simulink model "Encode_To_DC"  (Simulink 8.6)
settings: Solver=VariableStepAuto  StartTime=0.0  StopTime=inf  RelTol=1e-3
libraries: hdlsllib x30, simulink x26, dspnetwork x2
settings Model: Creator=Oscar  LastModifiedBy=Oscar
settings DataIOCC: SaveFormat=Dataset  SignalLoggingSaveFormat=Dataset
settings OptimizationCC: ExpressionDepthLimit=128
settings DebuggingCC: UnderspecifiedInitializationDetection=Simplified  MergeDetectMultiDrivingBlocksExec=error  SolverPrmCheckMsg=none  FcnCallInpInsideContextMsg=EnableAllAsError  StateNameClashWarn=none
settings HardwareCC: ProdBitPerPointer=64  ProdLargestAtomicFloat=Float  ProdIntDivRoundTo=Zero  ProdEndianess=LittleEndian  ProdWordSize=64  ProdHWDeviceType=Intel->x86-64 (Windows64)
settings GRTTargetCC: GeneratePreprocessorConditionals=Use local settings  CombineOutputUpdateFcns=on  GRTInterface=off
settings ConfigComp: CovModelRefEnable=off

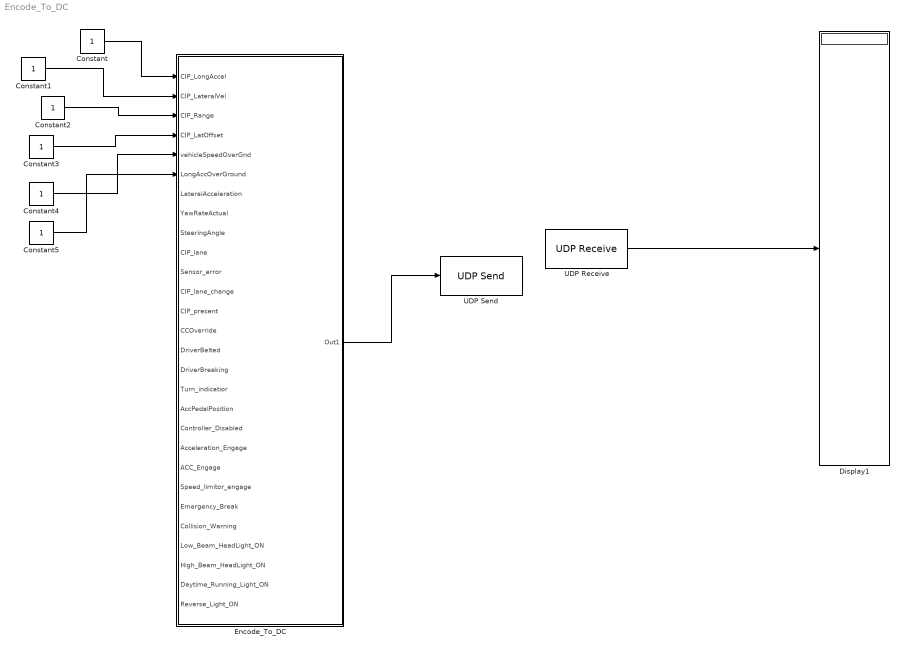
== system Encode_To_DC ==
  Constant{,1..5} (6 alike) : Constant
  Display1 : Display
      settings: Format=hex (Stored Integer)
  Encode_To_DC : Subsystem
  UDP Receive : dspnetwork/UDP Receive  localURL='0.0.0.0'  localPort=25000  remoteURL='localhost'  remotePort=-1  recvBufferSize=8192  dims=255  signalDatatype=uint16  isVarSize=on  showBlockingTime=off  blockingTime=0  sampletime=1
  UDP Send : dspnetwork/UDP Send  remoteURL='127.0.0.1'  remotePort=25000  localURL='0.0.0.0'  localPortSource=Automatically determine  localPort=-1  sampletime=-1  separateLengthPort=0
  wires:
  Encode_To_DC/1(Out1) -> UDP Send/1
  Constant/1 -> Encode_To_DC/1(CIP_LongAccel)
  UDP Receive/1 -> Display1/1
  Constant1/1 -> Encode_To_DC/2(CIP_LateralVel)
  Constant2/1 -> Encode_To_DC/3(CIP_Range)
  Constant3/1 -> Encode_To_DC/4(CIP_LatOffset)
  Constant4/1 -> Encode_To_DC/5(vehicleSpeedOverGnd)
  Constant5/1 -> Encode_To_DC/6(LongAccOverGround)

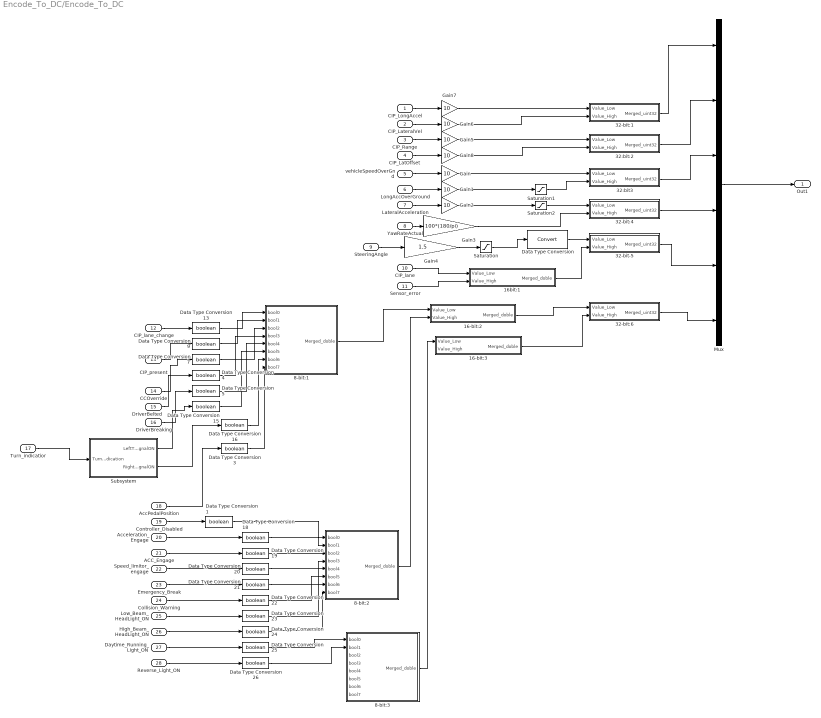
== system Encode_To_DC/Encode_To_DC ==
  CIP_LongAccel : Inport
  CIP_LateralVel : Inport  Port=2
  CIP_Range : Inport  Port=3
  CIP_LatOffset : Inport  Port=4
  vehicleSpeedOverGnd : Inport  Port=5
  LongAccOverGround : Inport  Port=6
  LateralAcceleration : Inport  Port=7
  YawRateActual : Inport  Port=8
  SteeringAngle : Inport  Port=9
  CIP_lane : Inport  Port=10
  Sensor_error : Inport  Port=11
  CIP_lane_change : Inport  Port=12
  CIP_present : Inport  Port=13
  CCOverride : Inport  Port=14
  DriverBelted : Inport  Port=15
  DriverBreaking : Inport  Port=16
  Turn_indicatior : Inport  Port=17
  AccPedalPosition : Inport  Port=18
  Controller_Disabled : Inport  Port=19
  Acceleration_Engage : Inport  Port=20
  ACC_Engage : Inport  Port=21
  Speed_limitor_engage : Inport  Port=22
  Emergency_Break : Inport  Port=23
  Collision_Warning : Inport  Port=24
  Low_Beam_HeadLight_ON : Inport  Port=25
  High_Beam_HeadLight_ON : Inport  Port=26
  Daytime_Running_Light_ON : Inport  Port=27
  Reverse_Light_ON : Inport  Port=28
  16-bit:2 : Subsystem
  16-bit:3 : Subsystem
  16bit:1 : Subsystem
  32-bit-5 : Subsystem
  32-bit:1 : Subsystem
  32-bit:4 : Subsystem
  32-bit:6 : Subsystem
  32:bit3 : Subsystem
  32:bit:2 : Subsystem
  8-bit:1 : Subsystem
  8-bit:2 : Subsystem
  8-bit:3 : Subsystem
  Data Type Conversion : DataTypeConversion
  Data Type Conversion{1,3..5,7,9,13,15..16,18..26} (18 alike) : DataTypeConversion  OutDataTypeStr=boolean  RndMeth=Nearest
  Gain{,1..2,5..8} (7 alike) : Gain  Gain=10
  Gain3 : Gain  Gain=100*(180/pi)
  Gain4 : Gain  Gain=1.5  OutMin=[-511]  OutMax=[512]  OutDataTypeStr=int16  SaturateOnIntegerOverflow=on
  Mux : Mux  Inputs=6
  Saturation : Saturate  UpperLimit=512  LowerLimit=-511
  Saturation1 : Saturate  UpperLimit=160  LowerLimit=-160
  Saturation2 : Saturate  UpperLimit=160  LowerLimit=-160
  Subsystem : Subsystem
  Out1 : Outport
  wires:
  LongAccOverGround/1 -> Gain1/1
  CIP_LateralVel/1 -> Gain6/1
  Turn_indicatior/1 -> Subsystem/1(Turn_Indication)
  DriverBreaking/1 -> Data Type Conversion5/1
  DriverBelted/1 -> Data Type Conversion4/1
  LateralAcceleration/1 -> Gain2/1
  CIP_lane_change/1 -> Data Type Conversion13/1
  AccPedalPosition/1 -> Data Type Conversion3/1
  CCOverride/1 -> Data Type Conversion7/1
  Mux/1 -> Out1/1
  CIP_present/1 -> Data Type Conversion9/1
  CIP_Range/1 -> Gain5/1
  Gain1/1 -> Saturation1/1
  Gain2/1 -> Saturation2/1
  Subsystem/1(LeftTurnSignalON) -> Data Type Conversion15/1
  Gain5/1 -> 32:bit:2/1(Value_Low)
  Gain6/1 -> 32-bit:1/2(Value_High)
  CIP_LongAccel/1 -> Gain7/1
  Gain7/1 -> 32-bit:1/1(Value_Low)
  CIP_LatOffset/1 -> Gain8/1
  Gain8/1 -> 32:bit:2/2(Value_High)
  Subsystem/2(RightTurnSignalON) -> Data Type Conversion16/1
  Controller_Disabled/1 -> Data Type Conversion1/1
  Acceleration_Engage/1 -> Data Type Conversion18/1
  ACC_Engage/1 -> Data Type Conversion19/1
  Speed_limitor_engage/1 -> Data Type Conversion20/1
  Emergency_Break/1 -> Data Type Conversion21/1
  Collision_Warning/1 -> Data Type Conversion22/1
  Low_Beam_HeadLight_ON/1 -> Data Type Conversion23/1
  High_Beam_HeadLight_ON/1 -> Data Type Conversion24/1
  Daytime_Running_Light_ON/1 -> Data Type Conversion25/1
  Reverse_Light_ON/1 -> Data Type Conversion26/1
  32-bit:1/1(Merged_uint32) -> Mux/1
  32:bit:2/1(Merged_uint32) -> Mux/2
  vehicleSpeedOverGnd/1 -> Gain/1
  Gain/1 -> 32:bit3/1(Value_Low)
  Saturation1/1 -> 32:bit3/2(Value_High)
  YawRateActual/1 -> Gain3/1
  SteeringAngle/1 -> Gain4/1
  Gain4/1 -> Saturation/1
  Saturation2/1 -> 32-bit:4/1(Value_Low)
  Gain3/1 -> 32-bit:4/2(Value_High)
  Saturation/1 -> Data Type Conversion/1
  32:bit3/1(Merged_uint32) -> Mux/3
  32-bit:4/1(Merged_uint32) -> Mux/4
  32-bit-5/1(Merged_uint32) -> Mux/5
  Data Type Conversion/1 -> 32-bit-5/1(Value_Low)
  CIP_lane/1 -> 16bit:1/1(Value_Low)
  Sensor_error/1 -> 16bit:1/2(Value_High)
  16bit:1/1(Merged_doble) -> 32-bit-5/2(Value_High)
  8-bit:1/1(Merged_doble) -> 16-bit:2/1(Value_Low)
  8-bit:2/1(Merged_doble) -> 16-bit:2/2(Value_High)
  32-bit:6/1(Merged_uint32) -> Mux/6
  16-bit:2/1(Merged_doble) -> 32-bit:6/1(Value_Low)
  Data Type Conversion13/1 -> 8-bit:1/1(bool0)
  Data Type Conversion9/1 -> 8-bit:1/2(bool1)
  Data Type Conversion7/1 -> 8-bit:1/3(bool2)
  Data Type Conversion4/1 -> 8-bit:1/4(bool3)
  Data Type Conversion5/1 -> 8-bit:1/5(bool4)
  Data Type Conversion15/1 -> 8-bit:1/6(bool5)
  Data Type Conversion16/1 -> 8-bit:1/7(bool6)
  Data Type Conversion3/1 -> 8-bit:1/8(bool7)
  Data Type Conversion1/1 -> 8-bit:2/1(bool0)
  Data Type Conversion18/1 -> 8-bit:2/2(bool1)
  Data Type Conversion19/1 -> 8-bit:2/3(bool2)
  Data Type Conversion20/1 -> 8-bit:2/4(bool3)
  Data Type Conversion21/1 -> 8-bit:2/5(bool4)
  Data Type Conversion22/1 -> 8-bit:2/6(bool5)
  Data Type Conversion23/1 -> 8-bit:2/7(bool6)
  Data Type Conversion24/1 -> 8-bit:2/8(bool7)
  8-bit:3/1(Merged_doble) -> 16-bit:3/1(Value_Low)
  Data Type Conversion25/1 -> 8-bit:3/1(bool0)
  Data Type Conversion26/1 -> 8-bit:3/2(bool1)
  16-bit:3/1(Merged_doble) -> 32-bit:6/2(Value_High)

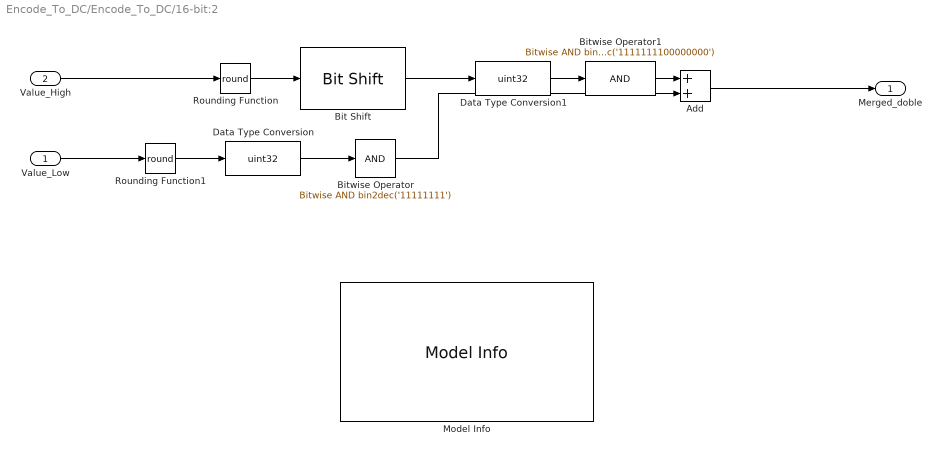
== system Encode_To_DC/Encode_To_DC/16-bit:2 ==
  Value_Low : Inport
  Value_High : Inport  Port=2
  Add : Sum  OutDataTypeStr=double
  Bit Shift : hdlsllib/HDL Operations/Bit Shift  mode=Shift Left Logical  N=8
  Bitwise Operator : simulink/Logic and Bit Operations/Bitwise Operator  logicop=AND  UseBitMask=on  BitMask=bin2dec('11111111')  BitMaskRealWorld=Stored Integer
  Bitwise Operator1 : simulink/Logic and Bit Operations/Bitwise Operator  logicop=AND  UseBitMask=on  BitMask=bin2dec('1111111100000000')  BitMaskRealWorld=Stored Integer
  Data Type Conversion : DataTypeConversion  OutDataTypeStr=uint32
  Data Type Conversion1 : DataTypeConversion  OutDataTypeStr=uint32
  Model Info : simulink/Model-Wide Utilities/Model Info  Frame=on  DisplayStringWithTags=|  HorizontalTextAlignment=Center  LeftAlignmentValue=0.5  SourceBlockDiagram=Encode_To_DC  TagMaxNumber=20
      | %<Created>
      | %<Creator>
      | 
      | Shift and round two double values into one double value.
      | 
      | input:	two double values (treated as 8-bit)
      | output:	One double value(treated as 16-bit)
  Rounding Function : Rounding  Operator=round
  Rounding Function1 : Rounding  Operator=round
  Merged_doble : Outport
  wires:
  Bit Shift/1 -> Data Type Conversion1/1
  Data Type Conversion1/1 -> Bitwise Operator1/1
  Rounding Function/1 -> Bit Shift/1
  Data Type Conversion/1 -> Bitwise Operator/1
  Bitwise Operator/1 -> Add/2
  Rounding Function1/1 -> Data Type Conversion/1
  Bitwise Operator1/1 -> Add/1
  Add/1 -> Merged_doble/1
  Value_Low/1 -> Rounding Function1/1
  Value_High/1 -> Rounding Function/1

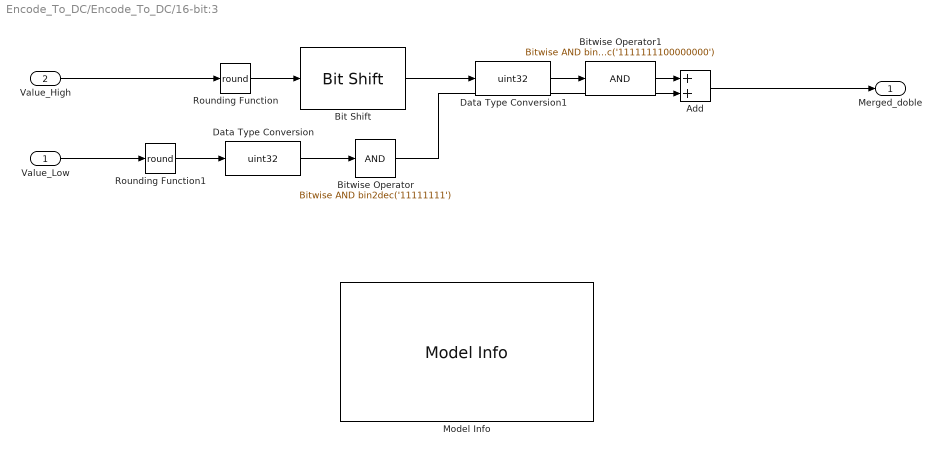
== system Encode_To_DC/Encode_To_DC/16-bit:3 ==
  Value_Low : Inport
  Value_High : Inport  Port=2
  Add : Sum  OutDataTypeStr=double
  Bit Shift : hdlsllib/HDL Operations/Bit Shift  mode=Shift Left Logical  N=8
  Bitwise Operator : simulink/Logic and Bit Operations/Bitwise Operator  logicop=AND  UseBitMask=on  BitMask=bin2dec('11111111')  BitMaskRealWorld=Stored Integer
  Bitwise Operator1 : simulink/Logic and Bit Operations/Bitwise Operator  logicop=AND  UseBitMask=on  BitMask=bin2dec('1111111100000000')  BitMaskRealWorld=Stored Integer
  Data Type Conversion : DataTypeConversion  OutDataTypeStr=uint32
  Data Type Conversion1 : DataTypeConversion  OutDataTypeStr=uint32
  Model Info : simulink/Model-Wide Utilities/Model Info  Frame=on  DisplayStringWithTags=|  HorizontalTextAlignment=Center  LeftAlignmentValue=0.5  SourceBlockDiagram=Encode_To_DC  TagMaxNumber=20
      | %<Created>
      | %<Creator>
      | 
      | Shift and round two double values into one double value.
      | 
      | input:	two double values (treated as 8-bit)
      | output:	One double value(treated as 16-bit)
  Rounding Function : Rounding  Operator=round
  Rounding Function1 : Rounding  Operator=round
  Merged_doble : Outport
  wires:
  Bit Shift/1 -> Data Type Conversion1/1
  Data Type Conversion1/1 -> Bitwise Operator1/1
  Rounding Function/1 -> Bit Shift/1
  Data Type Conversion/1 -> Bitwise Operator/1
  Bitwise Operator/1 -> Add/2
  Rounding Function1/1 -> Data Type Conversion/1
  Bitwise Operator1/1 -> Add/1
  Add/1 -> Merged_doble/1
  Value_Low/1 -> Rounding Function1/1
  Value_High/1 -> Rounding Function/1

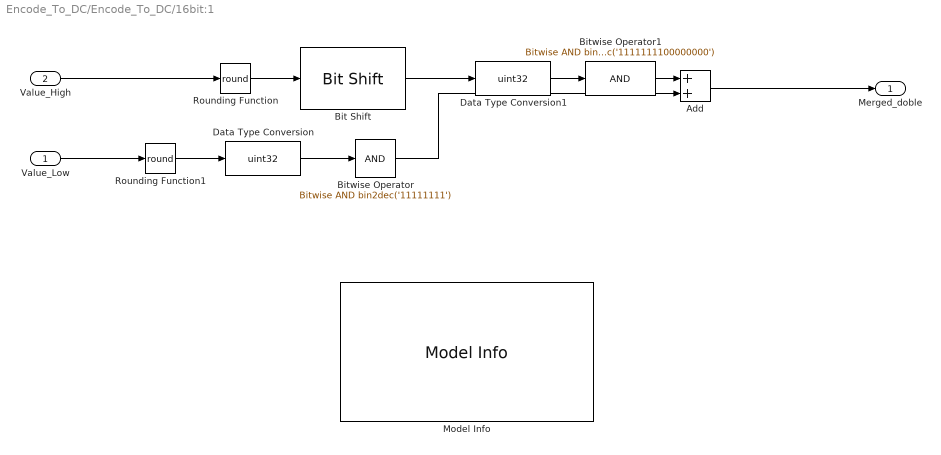
== system Encode_To_DC/Encode_To_DC/16bit:1 ==
  Value_Low : Inport
  Value_High : Inport  Port=2
  Add : Sum  OutDataTypeStr=double
  Bit Shift : hdlsllib/HDL Operations/Bit Shift  mode=Shift Left Logical  N=8
  Bitwise Operator : simulink/Logic and Bit Operations/Bitwise Operator  logicop=AND  UseBitMask=on  BitMask=bin2dec('11111111')  BitMaskRealWorld=Stored Integer
  Bitwise Operator1 : simulink/Logic and Bit Operations/Bitwise Operator  logicop=AND  UseBitMask=on  BitMask=bin2dec('1111111100000000')  BitMaskRealWorld=Stored Integer
  Data Type Conversion : DataTypeConversion  OutDataTypeStr=uint32
  Data Type Conversion1 : DataTypeConversion  OutDataTypeStr=uint32
  Model Info : simulink/Model-Wide Utilities/Model Info  Frame=on  DisplayStringWithTags=|  HorizontalTextAlignment=Center  LeftAlignmentValue=0.5  SourceBlockDiagram=Encode_To_DC  TagMaxNumber=20
      | %<Created>
      | %<Creator>
      | 
      | Shift and round two double values into one double value.
      | 
      | input:	two double values (treated as 8-bit)
      | output:	One double value(treated as 16-bit)
  Rounding Function : Rounding  Operator=round
  Rounding Function1 : Rounding  Operator=round
  Merged_doble : Outport
  wires:
  Bit Shift/1 -> Data Type Conversion1/1
  Data Type Conversion1/1 -> Bitwise Operator1/1
  Rounding Function/1 -> Bit Shift/1
  Data Type Conversion/1 -> Bitwise Operator/1
  Bitwise Operator/1 -> Add/2
  Rounding Function1/1 -> Data Type Conversion/1
  Bitwise Operator1/1 -> Add/1
  Add/1 -> Merged_doble/1
  Value_Low/1 -> Rounding Function1/1
  Value_High/1 -> Rounding Function/1

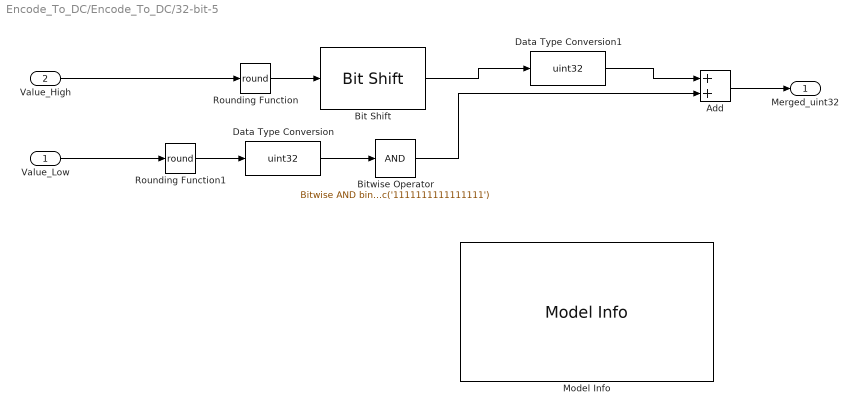
== system Encode_To_DC/Encode_To_DC/32-bit-5 ==
  Value_Low : Inport
  Value_High : Inport  Port=2
  Add : Sum
  Bit Shift : hdlsllib/HDL Operations/Bit Shift  mode=Shift Left Logical  N=16
  Bitwise Operator : simulink/Logic and Bit Operations/Bitwise Operator  logicop=AND  UseBitMask=on  BitMask=bin2dec('1111111111111111')  BitMaskRealWorld=Stored Integer
  Data Type Conversion : DataTypeConversion  OutDataTypeStr=uint32
  Data Type Conversion1 : DataTypeConversion  OutDataTypeStr=uint32
  Model Info : simulink/Model-Wide Utilities/Model Info  Frame=on  DisplayStringWithTags=|  HorizontalTextAlignment=Center  LeftAlignmentValue=0.5  SourceBlockDiagram=Encode_To_DC  TagMaxNumber=20
      | %<Created>
      | %<Creator>
      | 
      | Shift and round two double values into one double value.
      | 
      | input:	two double values (treated as 16-bit)
      | output:	One uint32 value
  Rounding Function : Rounding  Operator=round
  Rounding Function1 : Rounding  Operator=round
  Merged_uint32 : Outport
  wires:
  Bit Shift/1 -> Data Type Conversion1/1
  Data Type Conversion1/1 -> Add/1
  Rounding Function/1 -> Bit Shift/1
  Data Type Conversion/1 -> Bitwise Operator/1
  Add/1 -> Merged_uint32/1
  Bitwise Operator/1 -> Add/2
  Rounding Function1/1 -> Data Type Conversion/1
  Value_High/1 -> Rounding Function/1
  Value_Low/1 -> Rounding Function1/1

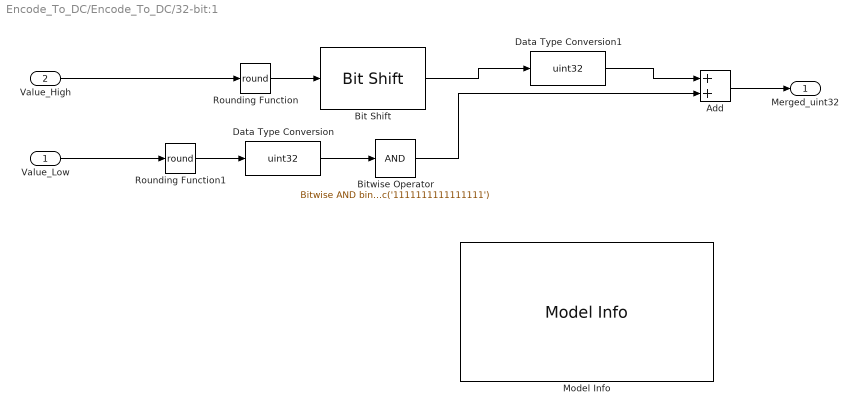
== system Encode_To_DC/Encode_To_DC/32-bit:1 ==
  Value_Low : Inport
  Value_High : Inport  Port=2
  Add : Sum
  Bit Shift : hdlsllib/HDL Operations/Bit Shift  mode=Shift Left Logical  N=16
  Bitwise Operator : simulink/Logic and Bit Operations/Bitwise Operator  logicop=AND  UseBitMask=on  BitMask=bin2dec('1111111111111111')  BitMaskRealWorld=Stored Integer
  Data Type Conversion : DataTypeConversion  OutDataTypeStr=uint32
  Data Type Conversion1 : DataTypeConversion  OutDataTypeStr=uint32
  Model Info : simulink/Model-Wide Utilities/Model Info  Frame=on  DisplayStringWithTags=|  HorizontalTextAlignment=Center  LeftAlignmentValue=0.5  SourceBlockDiagram=Encode_To_DC  TagMaxNumber=20
      | %<Created>
      | %<Creator>
      | 
      | Shift and round two double values into one double value.
      | 
      | input:	two double values (treated as 16-bit)
      | output:	One uint32 value
  Rounding Function : Rounding  Operator=round
  Rounding Function1 : Rounding  Operator=round
  Merged_uint32 : Outport
  wires:
  Bit Shift/1 -> Data Type Conversion1/1
  Data Type Conversion1/1 -> Add/1
  Rounding Function/1 -> Bit Shift/1
  Data Type Conversion/1 -> Bitwise Operator/1
  Add/1 -> Merged_uint32/1
  Bitwise Operator/1 -> Add/2
  Rounding Function1/1 -> Data Type Conversion/1
  Value_High/1 -> Rounding Function/1
  Value_Low/1 -> Rounding Function1/1

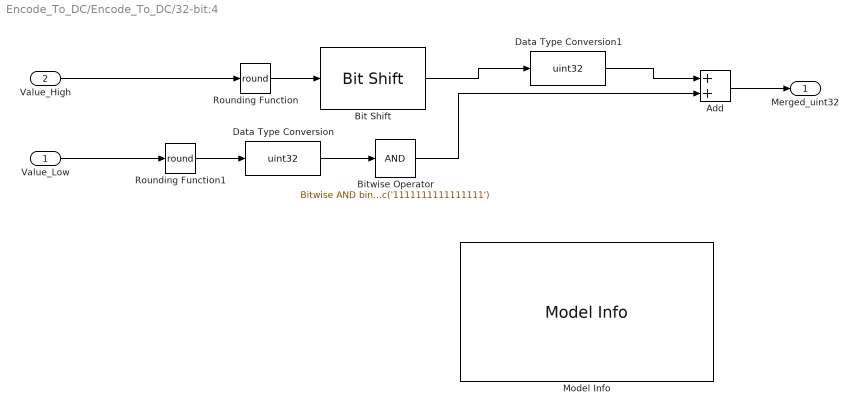
== system Encode_To_DC/Encode_To_DC/32-bit:4 ==
  Value_Low : Inport
  Value_High : Inport  Port=2
  Add : Sum
  Bit Shift : hdlsllib/HDL Operations/Bit Shift  mode=Shift Left Logical  N=16
  Bitwise Operator : simulink/Logic and Bit Operations/Bitwise Operator  logicop=AND  UseBitMask=on  BitMask=bin2dec('1111111111111111')  BitMaskRealWorld=Stored Integer
  Data Type Conversion : DataTypeConversion  OutDataTypeStr=uint32
  Data Type Conversion1 : DataTypeConversion  OutDataTypeStr=uint32
  Model Info : simulink/Model-Wide Utilities/Model Info  Frame=on  DisplayStringWithTags=|  HorizontalTextAlignment=Center  LeftAlignmentValue=0.5  SourceBlockDiagram=Encode_To_DC  TagMaxNumber=20
      | %<Created>
      | %<Creator>
      | 
      | Shift and round two double values into one double value.
      | 
      | input:	two double values (treated as 16-bit)
      | output:	One uint32 value
  Rounding Function : Rounding  Operator=round
  Rounding Function1 : Rounding  Operator=round
  Merged_uint32 : Outport
  wires:
  Bit Shift/1 -> Data Type Conversion1/1
  Data Type Conversion1/1 -> Add/1
  Rounding Function/1 -> Bit Shift/1
  Data Type Conversion/1 -> Bitwise Operator/1
  Add/1 -> Merged_uint32/1
  Bitwise Operator/1 -> Add/2
  Rounding Function1/1 -> Data Type Conversion/1
  Value_High/1 -> Rounding Function/1
  Value_Low/1 -> Rounding Function1/1

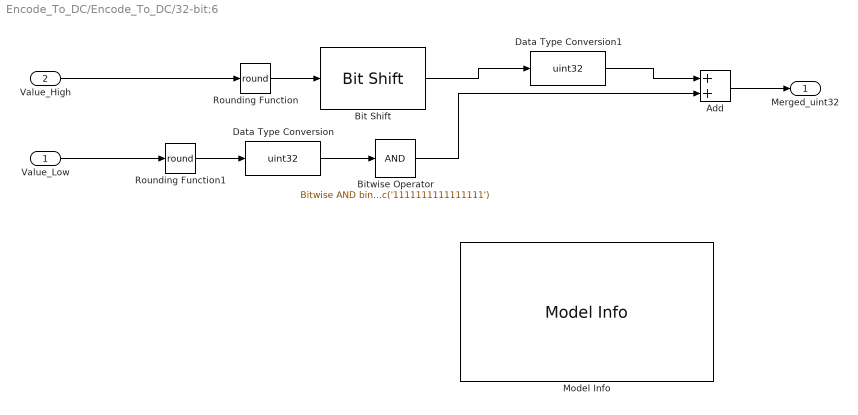
== system Encode_To_DC/Encode_To_DC/32-bit:6 ==
  Value_Low : Inport
  Value_High : Inport  Port=2
  Add : Sum
  Bit Shift : hdlsllib/HDL Operations/Bit Shift  mode=Shift Left Logical  N=16
  Bitwise Operator : simulink/Logic and Bit Operations/Bitwise Operator  logicop=AND  UseBitMask=on  BitMask=bin2dec('1111111111111111')  BitMaskRealWorld=Stored Integer
  Data Type Conversion : DataTypeConversion  OutDataTypeStr=uint32
  Data Type Conversion1 : DataTypeConversion  OutDataTypeStr=uint32
  Model Info : simulink/Model-Wide Utilities/Model Info  Frame=on  DisplayStringWithTags=|  HorizontalTextAlignment=Center  LeftAlignmentValue=0.5  SourceBlockDiagram=Encode_To_DC  TagMaxNumber=20
      | %<Created>
      | %<Creator>
      | 
      | Shift and round two double values into one double value.
      | 
      | input:	two double values (treated as 16-bit)
      | output:	One uint32 value
  Rounding Function : Rounding  Operator=round
  Rounding Function1 : Rounding  Operator=round
  Merged_uint32 : Outport
  wires:
  Bit Shift/1 -> Data Type Conversion1/1
  Data Type Conversion1/1 -> Add/1
  Rounding Function/1 -> Bit Shift/1
  Data Type Conversion/1 -> Bitwise Operator/1
  Add/1 -> Merged_uint32/1
  Bitwise Operator/1 -> Add/2
  Rounding Function1/1 -> Data Type Conversion/1
  Value_High/1 -> Rounding Function/1
  Value_Low/1 -> Rounding Function1/1

== system Encode_To_DC/Encode_To_DC/32:bit3 ==
  Value_Low : Inport
  Value_High : Inport  Port=2
  Add : Sum
  Bit Shift : hdlsllib/HDL Operations/Bit Shift  mode=Shift Left Logical  N=16
  Bitwise Operator : simulink/Logic and Bit Operations/Bitwise Operator  logicop=AND  UseBitMask=on  BitMask=bin2dec('1111111111111111')  BitMaskRealWorld=Stored Integer
  Data Type Conversion : DataTypeConversion  OutDataTypeStr=uint32
  Data Type Conversion1 : DataTypeConversion  OutDataTypeStr=uint32
  Model Info : simulink/Model-Wide Utilities/Model Info  Frame=on  DisplayStringWithTags=|  HorizontalTextAlignment=Center  LeftAlignmentValue=0.5  SourceBlockDiagram=Encode_To_DC  TagMaxNumber=20
      | %<Created>
      | %<Creator>
      | 
      | Shift and round two double values into one double value.
      | 
      | input:	two double values (treated as 16-bit)
      | output:	One uint32 value
  Rounding Function : Rounding  Operator=round
  Rounding Function1 : Rounding  Operator=round
  Merged_uint32 : Outport
  wires:
  Bit Shift/1 -> Data Type Conversion1/1
  Data Type Conversion1/1 -> Add/1
  Rounding Function/1 -> Bit Shift/1
  Data Type Conversion/1 -> Bitwise Operator/1
  Add/1 -> Merged_uint32/1
  Bitwise Operator/1 -> Add/2
  Rounding Function1/1 -> Data Type Conversion/1
  Value_High/1 -> Rounding Function/1
  Value_Low/1 -> Rounding Function1/1

== system Encode_To_DC/Encode_To_DC/32:bit:2 ==
  Value_Low : Inport
  Value_High : Inport  Port=2
  Add : Sum
  Bit Shift : hdlsllib/HDL Operations/Bit Shift  mode=Shift Left Logical  N=16
  Bitwise Operator : simulink/Logic and Bit Operations/Bitwise Operator  logicop=AND  UseBitMask=on  BitMask=bin2dec('1111111111111111')  BitMaskRealWorld=Stored Integer
  Data Type Conversion : DataTypeConversion  OutDataTypeStr=uint32
  Data Type Conversion1 : DataTypeConversion  OutDataTypeStr=uint32
  Model Info : simulink/Model-Wide Utilities/Model Info  Frame=on  DisplayStringWithTags=|  HorizontalTextAlignment=Center  LeftAlignmentValue=0.5  SourceBlockDiagram=Encode_To_DC  TagMaxNumber=20
      | %<Created>
      | %<Creator>
      | 
      | Shift and round two double values into one double value.
      | 
      | input:	two double values (treated as 16-bit)
      | output:	One uint32 value
  Rounding Function : Rounding  Operator=round
  Rounding Function1 : Rounding  Operator=round
  Merged_uint32 : Outport
  wires:
  Bit Shift/1 -> Data Type Conversion1/1
  Data Type Conversion1/1 -> Add/1
  Rounding Function/1 -> Bit Shift/1
  Data Type Conversion/1 -> Bitwise Operator/1
  Add/1 -> Merged_uint32/1
  Bitwise Operator/1 -> Add/2
  Rounding Function1/1 -> Data Type Conversion/1
  Value_High/1 -> Rounding Function/1
  Value_Low/1 -> Rounding Function1/1

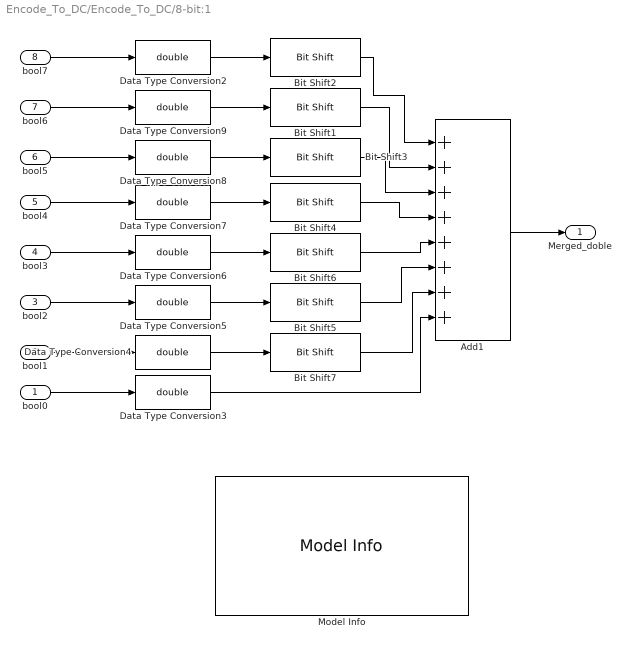
== system Encode_To_DC/Encode_To_DC/8-bit:1 ==
  bool0 : Inport
  bool1 : Inport  Port=2
  bool2 : Inport  Port=3
  bool3 : Inport  Port=4
  bool4 : Inport  Port=5
  bool5 : Inport  Port=6
  bool6 : Inport  Port=7
  bool7 : Inport  Port=8
  Add1 : Sum  Inputs=++++++++  OutDataTypeStr=double
  Bit Shift1 : hdlsllib/HDL Operations/Bit Shift  mode=Shift Left Logical  N=6
  Bit Shift2 : hdlsllib/HDL Operations/Bit Shift  mode=Shift Left Logical  N=7
  Bit Shift3 : hdlsllib/HDL Operations/Bit Shift  mode=Shift Left Logical  N=5
  Bit Shift4 : hdlsllib/HDL Operations/Bit Shift  mode=Shift Left Logical  N=4
  Bit Shift5 : hdlsllib/HDL Operations/Bit Shift  mode=Shift Left Logical  N=2
  Bit Shift6 : hdlsllib/HDL Operations/Bit Shift  mode=Shift Left Logical  N=3
  Bit Shift7 : hdlsllib/HDL Operations/Bit Shift  mode=Shift Left Logical  N=1
  Data Type Conversion{2..9} (8 alike) : DataTypeConversion  OutDataTypeStr=double
  Model Info : simulink/Model-Wide Utilities/Model Info  Frame=on  DisplayStringWithTags=|  HorizontalTextAlignment=Center  LeftAlignmentValue=0.5  SourceBlockDiagram=Encode_To_DC  TagMaxNumber=20
      | %<Created>
      | %<Creator>
      | 
      | Shift and round eight double values into one double value.
      | 
      | input:	Eight boolean values
      | output:	One double value(treated as 8-bit)
  Merged_doble : Outport
  wires:
  bool7/1 -> Data Type Conversion2/1
  Data Type Conversion2/1 -> Bit Shift2/1
  Bit Shift2/1 -> Add1/1
  Bit Shift1/1 -> Add1/2
  Bit Shift3/1 -> Add1/3
  Bit Shift4/1 -> Add1/4
  Bit Shift6/1 -> Add1/5
  Bit Shift5/1 -> Add1/6
  Bit Shift7/1 -> Add1/7
  Data Type Conversion3/1 -> Add1/8
  bool0/1 -> Data Type Conversion3/1
  Data Type Conversion4/1 -> Bit Shift7/1
  Data Type Conversion9/1 -> Bit Shift1/1
  Data Type Conversion8/1 -> Bit Shift3/1
  Data Type Conversion7/1 -> Bit Shift4/1
  Data Type Conversion6/1 -> Bit Shift6/1
  Data Type Conversion5/1 -> Bit Shift5/1
  bool1/1 -> Data Type Conversion4/1
  bool2/1 -> Data Type Conversion5/1
  bool3/1 -> Data Type Conversion6/1
  bool4/1 -> Data Type Conversion7/1
  bool5/1 -> Data Type Conversion8/1
  bool6/1 -> Data Type Conversion9/1
  Add1/1 -> Merged_doble/1

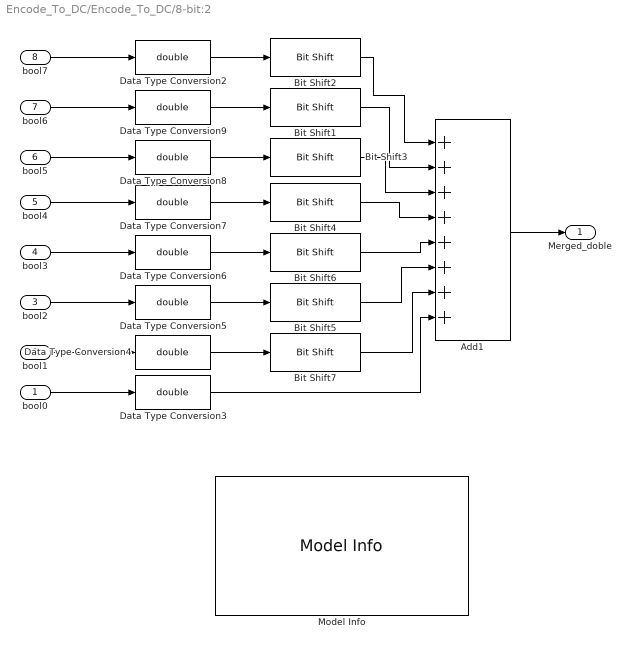
== system Encode_To_DC/Encode_To_DC/8-bit:2 ==
  bool0 : Inport
  bool1 : Inport  Port=2
  bool2 : Inport  Port=3
  bool3 : Inport  Port=4
  bool4 : Inport  Port=5
  bool5 : Inport  Port=6
  bool6 : Inport  Port=7
  bool7 : Inport  Port=8
  Add1 : Sum  Inputs=++++++++  OutDataTypeStr=double
  Bit Shift1 : hdlsllib/HDL Operations/Bit Shift  mode=Shift Left Logical  N=6
  Bit Shift2 : hdlsllib/HDL Operations/Bit Shift  mode=Shift Left Logical  N=7
  Bit Shift3 : hdlsllib/HDL Operations/Bit Shift  mode=Shift Left Logical  N=5
  Bit Shift4 : hdlsllib/HDL Operations/Bit Shift  mode=Shift Left Logical  N=4
  Bit Shift5 : hdlsllib/HDL Operations/Bit Shift  mode=Shift Left Logical  N=2
  Bit Shift6 : hdlsllib/HDL Operations/Bit Shift  mode=Shift Left Logical  N=3
  Bit Shift7 : hdlsllib/HDL Operations/Bit Shift  mode=Shift Left Logical  N=1
  Data Type Conversion{2..9} (8 alike) : DataTypeConversion  OutDataTypeStr=double
  Model Info : simulink/Model-Wide Utilities/Model Info  Frame=on  DisplayStringWithTags=|  HorizontalTextAlignment=Center  LeftAlignmentValue=0.5  SourceBlockDiagram=Encode_To_DC  TagMaxNumber=20
      | %<Created>
      | %<Creator>
      | 
      | Shift and round eight double values into one double value.
      | 
      | input:	Eight boolean values
      | output:	One double value(treated as 8-bit)
  Merged_doble : Outport
  wires:
  bool7/1 -> Data Type Conversion2/1
  Data Type Conversion2/1 -> Bit Shift2/1
  Bit Shift2/1 -> Add1/1
  Bit Shift1/1 -> Add1/2
  Bit Shift3/1 -> Add1/3
  Bit Shift4/1 -> Add1/4
  Bit Shift6/1 -> Add1/5
  Bit Shift5/1 -> Add1/6
  Bit Shift7/1 -> Add1/7
  Data Type Conversion3/1 -> Add1/8
  bool0/1 -> Data Type Conversion3/1
  Data Type Conversion4/1 -> Bit Shift7/1
  Data Type Conversion9/1 -> Bit Shift1/1
  Data Type Conversion8/1 -> Bit Shift3/1
  Data Type Conversion7/1 -> Bit Shift4/1
  Data Type Conversion6/1 -> Bit Shift6/1
  Data Type Conversion5/1 -> Bit Shift5/1
  bool1/1 -> Data Type Conversion4/1
  bool2/1 -> Data Type Conversion5/1
  bool3/1 -> Data Type Conversion6/1
  bool4/1 -> Data Type Conversion7/1
  bool5/1 -> Data Type Conversion8/1
  bool6/1 -> Data Type Conversion9/1
  Add1/1 -> Merged_doble/1

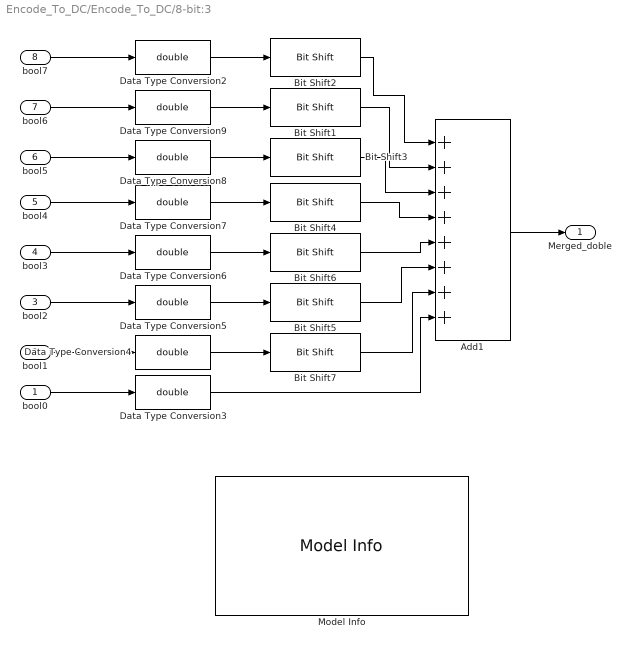
== system Encode_To_DC/Encode_To_DC/8-bit:3 ==
  bool0 : Inport
  bool1 : Inport  Port=2
  bool2 : Inport  Port=3
  bool3 : Inport  Port=4
  bool4 : Inport  Port=5
  bool5 : Inport  Port=6
  bool6 : Inport  Port=7
  bool7 : Inport  Port=8
  Add1 : Sum  Inputs=++++++++  OutDataTypeStr=double
  Bit Shift1 : hdlsllib/HDL Operations/Bit Shift  mode=Shift Left Logical  N=6
  Bit Shift2 : hdlsllib/HDL Operations/Bit Shift  mode=Shift Left Logical  N=7
  Bit Shift3 : hdlsllib/HDL Operations/Bit Shift  mode=Shift Left Logical  N=5
  Bit Shift4 : hdlsllib/HDL Operations/Bit Shift  mode=Shift Left Logical  N=4
  Bit Shift5 : hdlsllib/HDL Operations/Bit Shift  mode=Shift Left Logical  N=2
  Bit Shift6 : hdlsllib/HDL Operations/Bit Shift  mode=Shift Left Logical  N=3
  Bit Shift7 : hdlsllib/HDL Operations/Bit Shift  mode=Shift Left Logical  N=1
  Data Type Conversion{2..9} (8 alike) : DataTypeConversion  OutDataTypeStr=double
  Model Info : simulink/Model-Wide Utilities/Model Info  Frame=on  DisplayStringWithTags=|  HorizontalTextAlignment=Center  LeftAlignmentValue=0.5  SourceBlockDiagram=Encode_To_DC  TagMaxNumber=20
      | %<Created>
      | %<Creator>
      | 
      | Shift and round eight double values into one double value.
      | 
      | input:	Eight boolean values
      | output:	One double value(treated as 8-bit)
  Merged_doble : Outport
  wires:
  bool7/1 -> Data Type Conversion2/1
  Data Type Conversion2/1 -> Bit Shift2/1
  Bit Shift2/1 -> Add1/1
  Bit Shift1/1 -> Add1/2
  Bit Shift3/1 -> Add1/3
  Bit Shift4/1 -> Add1/4
  Bit Shift6/1 -> Add1/5
  Bit Shift5/1 -> Add1/6
  Bit Shift7/1 -> Add1/7
  Data Type Conversion3/1 -> Add1/8
  bool0/1 -> Data Type Conversion3/1
  Data Type Conversion4/1 -> Bit Shift7/1
  Data Type Conversion9/1 -> Bit Shift1/1
  Data Type Conversion8/1 -> Bit Shift3/1
  Data Type Conversion7/1 -> Bit Shift4/1
  Data Type Conversion6/1 -> Bit Shift6/1
  Data Type Conversion5/1 -> Bit Shift5/1
  bool1/1 -> Data Type Conversion4/1
  bool2/1 -> Data Type Conversion5/1
  bool3/1 -> Data Type Conversion6/1
  bool4/1 -> Data Type Conversion7/1
  bool5/1 -> Data Type Conversion8/1
  bool6/1 -> Data Type Conversion9/1
  Add1/1 -> Merged_doble/1

== system Encode_To_DC/Encode_To_DC/Subsystem ==
  Turn_Indication : Inport
  Left : simulink/Logic and Bit Operations/Compare To Constant  relop===  const=1  OutDataTypeStr=boolean
  Right : simulink/Logic and Bit Operations/Compare To Constant  relop===  const=2  OutDataTypeStr=boolean
  LeftTurnSignalON : Outport
  RightTurnSignalON : Outport  Port=2
  wires:
  Turn_Indication/1 -> Right/1, Left/1
  Left/1 -> LeftTurnSignalON/1
  Right/1 -> RightTurnSignalON/1
